simulink library "simpleTetheredBalloon"  (R2020a)
settings: Solver=VariableStepAuto  StartTime=0.0  StopTime=10.0  RelTol=1e-3
libraries: vrlib x2
settings Model: Creator=Ayaz  LastModifiedBy=Ayaz

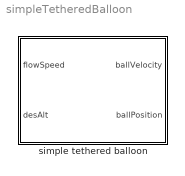
== system simpleTetheredBalloon ==
  simple tethered balloon : Subsystem  mask{rhoEnv=1.225, rhoBall=1, rBall=10, cdBall=.5, kSpring=5e6, iniAlt=600, kp=1, ki=0.1, tau=1}
      mask prompts: rhoEnv "Environment density [kg/m^3]"; rhoBall "Balloon density [kg/m^3]"; rBall "Balloon radius [m]"; cdBall "Balloon drag coefficient"; kSpring "Tether sping constant"; iniAlt "Initial altitude"; kp "Proportional gain [(m/s)/m]"; ki "Intergral gain [(m/s)/(m*s)]"; tau "Time constant"
      mask DialogControl Container3 Prompt: Altitude controller

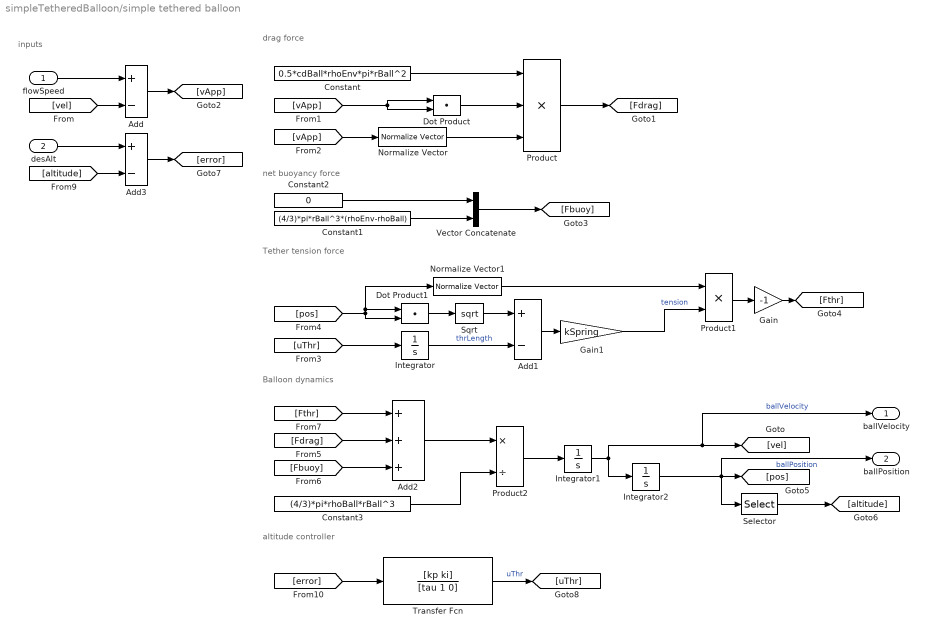
== system simpleTetheredBalloon/simple tethered balloon ==
  note: Balloon dynamics
  note: altitude controller
  note: inputs
  note: Tether tension force
  note: net buoyancy force
  note: drag force
  flowSpeed : Inport
  desAlt : Inport  Port=2
  Add : Sum  Inputs=+-
  Add1 : Sum  Inputs=+-
  Add2 : Sum  Inputs=+++
  Add3 : Sum  Inputs=+-
  Constant : Constant  Value=0.5*cdBall*rhoEnv*pi*rBall^2
  Constant1 : Constant  Value=(4/3)*pi*rBall^3*(rhoEnv-rhoBall)
  Constant2 : Constant  Value=0
  Constant3 : Constant  Value=(4/3)*pi*rhoBall*rBall^3
  Dot Product : DotProduct  InputSameDT=on  OutDataTypeStr=Inherit: Inherit via internal rule
  Dot Product1 : DotProduct  InputSameDT=on  OutDataTypeStr=Inherit: Inherit via internal rule
  Gain : Gain  Gain=-1
  Gain1 : Gain  Gain=kSpring
  Integrator : Integrator  InitialCondition=iniAlt
  Integrator1 : Integrator  InitialCondition=[0;0]
  Integrator2 : Integrator  InitialCondition=[0;iniAlt]
  Normalize Vector : vrlib/Utilities/Normalize Vector  maxzero=0
  Normalize Vector1 : vrlib/Utilities/Normalize Vector  maxzero=0
  Product : Product  Inputs=3
  Product1 : Product
  Product2 : Product  Inputs=*/
  Selector : Selector  InputPortWidth=2  IndexOptions=Index vector (dialog)  Indices=2  OutputSizes=1
  Sqrt : Sqrt  SaturateOnIntegerOverflow=on
  Transfer Fcn : TransferFcn  Numerator=[kp ki]  Denominator=[tau 1 0]
  Vector Concatenate : Concatenate
  ballVelocity : Outport
  ballPosition : Outport  Port=2
  wires:
  flowSpeed/1 -> Add/1
  [vel] -> Add/2
  Add/1 -> [vApp]
  [vApp] -> Dot Product/1, Dot Product/2
  [vApp] -> Normalize Vector/1
  Constant/1 -> Product/1
  Dot Product/1 -> Product/2
  Normalize Vector/1 -> Product/3
  Product/1 -> [Fdrag]
  Constant1/1 -> Vector Concatenate/2
  Constant2/1 -> Vector Concatenate/1
  Vector Concatenate/1 -> [Fbuoy]
  Dot Product1/1 -> Sqrt/1
  [pos] -> Dot Product1/1, Normalize Vector1/1, Dot Product1/2
  Sqrt/1 -> Add1/1
  Integrator/1 -> Add1/2  "thrLength"
  Normalize Vector1/1 -> Product1/1
  Add1/1 -> Gain1/1
  Product1/1 -> Gain/1
  Gain/1 -> [Fthr]
  [uThr] -> Integrator/1
  [Fthr] -> Add2/1
  [Fdrag] -> Add2/2
  [Fbuoy] -> Add2/3
  Add2/1 -> Product2/1
  Product2/1 -> Integrator1/1
  Constant3/1 -> Product2/2
  Integrator1/1 -> Integrator2/1, ballVelocity/1, [vel]  "ballVelocity"
  Integrator2/1 -> ballPosition/1, Selector/1, [pos]  "ballPosition"
  desAlt/1 -> Add3/1
  Selector/1 -> [altitude]
  [altitude] -> Add3/2
  Add3/1 -> [error]
  [error] -> Transfer Fcn/1
  Transfer Fcn/1 -> [uThr]  "uThr"
  Gain1/1 -> Product1/2  "tension"
